simulink model "sumpModel"  (R2019a)
settings: Solver=VariableStepAuto  StartTime=0.0  StopTime=10.0  RelTol=1e-3
settings Model: Creator=jason.miskin  LastModifiedBy=jason.miskin
settings DataIOCC: ExternalInput=[t, u1,u2,u3,u3]  LoadExternalInput=on

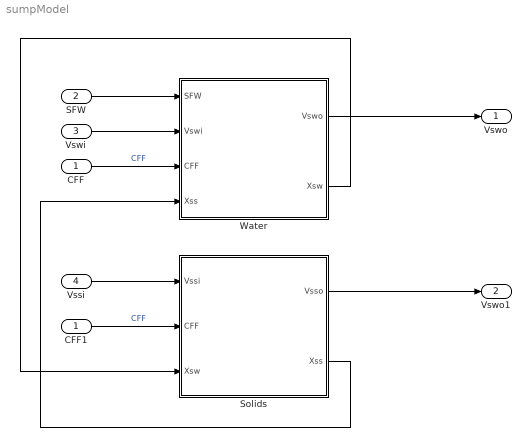
== system sumpModel ==
  CFF : Inport
  SFW : Inport  Port=2
  Vswi : Inport  Port=3
  Vssi : Inport  Port=4
  CFF1 : InportShadow
  Solids : Subsystem
  Water : Subsystem
  Vswo : Outport
  Vswo1 : Outport  Port=2
  wires:
  SFW/1 -> Water/1(SFW)
  Vswi/1 -> Water/2(Vswi)
  CFF/1 -> Water/3(CFF)  "CFF"
  Water/1(Vswo) -> Vswo/1
  Solids/1(Vsso) -> Vswo1/1
  Vssi/1 -> Solids/1(Vssi)
  CFF1/1 -> Solids/2(CFF)  "CFF"
  Solids/2(Xss) -> Water/4(Xss)
  Water/2(Xsw) -> Solids/3(Xsw)

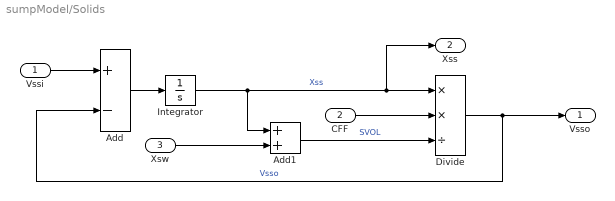
== system sumpModel/Solids ==
  Vssi : Inport
  CFF : Inport  Port=2
  Xsw : Inport  Port=3
  Add : Sum  Inputs=+-
  Add1 : Sum
  Divide : Product  Inputs=**/
  Integrator : Integrator  InitialCondition=15
  Vsso : Outport
  Xss : Outport  Port=2
  wires:
  CFF/1 -> Divide/2
  Vssi/1 -> Add/1
  Xsw/1 -> Add1/2
  Divide/1 -> Add/2, Vsso/1  "Vsso"
  Add/1 -> Integrator/1
  Add1/1 -> Divide/3  "SVOL"
  Integrator/1 -> Xss/1, Divide/1, Add1/1  "Xss"

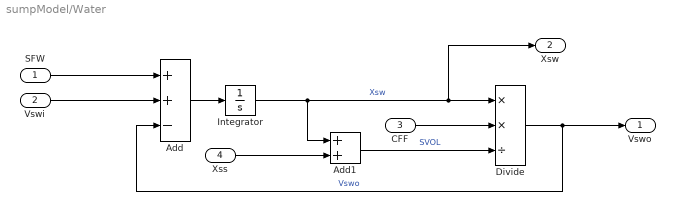
== system sumpModel/Water ==
  SFW : Inport
  Vswi : Inport  Port=2
  CFF : Inport  Port=3
  Xss : Inport  Port=4
  Add : Sum  Inputs=++-
  Add1 : Sum
  Divide : Product  Inputs=**/
  Integrator : Integrator  InitialCondition=15
  Vswo : Outport
  Xsw : Outport  Port=2
  wires:
  Integrator/1 -> Add1/1, Xsw/1, Divide/1  "Xsw"
  Add1/1 -> Divide/3  "SVOL"
  Add/1 -> Integrator/1
  Divide/1 -> Vswo/1, Add/3  "Vswo"
  Xss/1 -> Add1/2
  SFW/1 -> Add/1
  Vswi/1 -> Add/2
  CFF/1 -> Divide/2
